simulink model "PIControlWithObserverR2_discrete_reorder_fixedpt"  (R2022b)
settings: Solver=VariableStepAuto  StartTime=0.0  StopTime=Tsim  FixedStep=dTMax  MaxStep=dTMax  RelTol=1e-3
values from neighbouring files (symbols this model uses):
  A = [A11 A12;A21 A22]    [VmPIWithObserverDriver_02Dec2022.m]    (also in observer_coeff.m)
  a1 = -1    [VmPIWithObserverDriver_02Dec2022.m]    (also in pi_controller_coeff.m = 0)
  a2 = 0    [VmPIWithObserverDriver_02Dec2022.m]
  Adp = LdC_inv*Ad    [VmPIWithObserverDriver_02Dec2022.m]    (also in observer_coeff.m = Adp)
  B = [B11;B21]    [VmPIWithObserverDriver_02Dec2022.m]    (also in observer_coeff.m)
  b0 = Gcd.num{1}(1)    [VmPIWithObserverDriver_02Dec2022.m]    (also in pi_controller_coeff.m = 1)
  b1 = Gcd.num{1}(2)    [VmPIWithObserverDriver_02Dec2022.m]    (also in pi_controller_coeff.m = 0)
  b2 = 0    [VmPIWithObserverDriver_02Dec2022.m]
  Bdp = Bdp/dac_scale    [VmPIWithObserverDriver_02Dec2022.m]    (also in observer_coeff.m = Bdp/dac_scale*total_scale)
  C = [C11 C12;C21 C22;C31 C32]    [VmPIWithObserverDriver_02Dec2022.m]    (also in observer_coeff.m)
  D = zeros(3,1)    [VmPIWithObserverDriver_02Dec2022.m]    (also in observer_coeff.m)
  dac_scale = 2^15    (= 32768)    [VmPIWithObserverDriver_02Dec2022.m]
  Im_scale = dn_per_amp    (= 246419753.086)    [VmPIWithObserverDriver_02Dec2022.m]
  Ldp = Ldp*[1/Im_scale, 0; 0, 1/VP1_scale]    [VmPIWithObserverDriver_02Dec2022.m]    (also in observer_coeff.m = Ldp*[1/Im_scale, 0; 0, 1/VP1_scale]*total_scale)
  N = 3    [VmPIWithObserverDriver_02Dec2022.m]
  Ts = 1/(MSPS*1e6)    (= 4e-07)    [VmPIWithObserverDriver_02Dec2022.m]
  VmDes = 0.025    [VmPIWithObserverDriver_02Dec2022.m]
  VP1_scale = dn_per_volt*10*1.7    (= 222822.4)    [VmPIWithObserverDriver_02Dec2022.m]
  x0 = [0.1*VmDes 0]'    [VmPIWithObserverDriver_02Dec2022.m]
settings Model: Creator=seco6437  LastModifiedBy=delg
settings DebuggingCC: UnconnectedInputMsg=warning  UnconnectedOutputMsg=warning  UnconnectedLineMsg=warning
settings ModelReferenceCC: EnableRefExpFcnMdlSchedulingChecks=on
settings RTWCC: DLArmComputeVersion=19.05

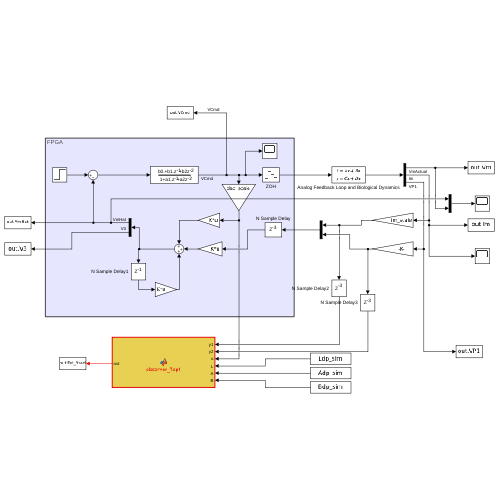
[thumbnail: Simulink's stored preview of the top-level diagram]
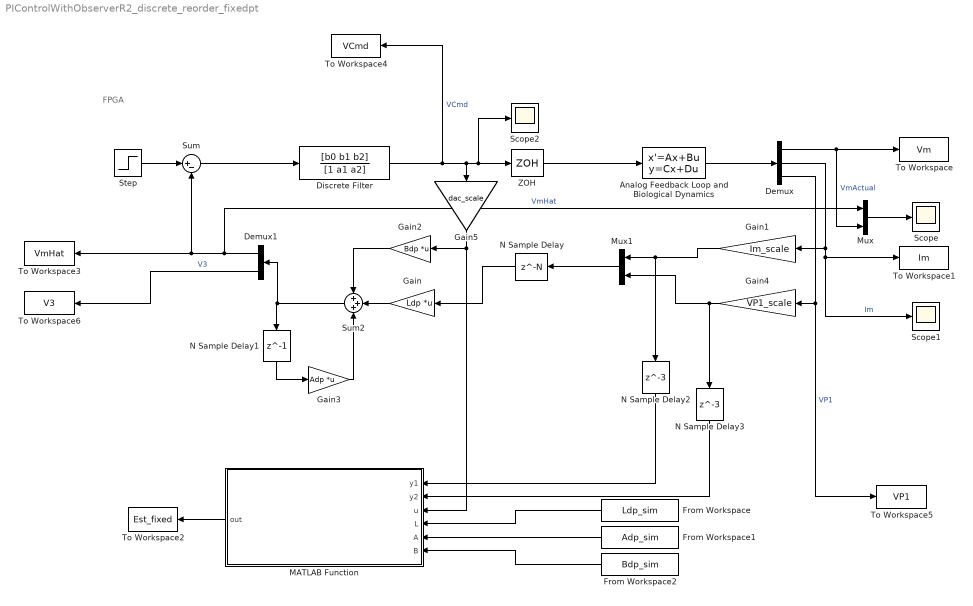
== system PIControlWithObserverR2_discrete_reorder_fixedpt ==
  note: FPGA
  Analog Feedback Loop and Biological Dynamics : StateSpace  A=A  B=B  C=C  D=D  InitialCondition=x0
  Demux : Demux  Outputs=3
  Demux1 : Demux  Outputs=2
  Discrete Filter : DiscreteFilter  Numerator=[b0 b1 b2]  Denominator=[1 a1 a2]  SampleTime=Ts
  From Workspace : FromWorkspace  VariableName=Ldp_sim  SampleTime=Ts  Interpolate=off  ZeroCross=off  OutputAfterFinalValue=Holding final value
  From Workspace1 : FromWorkspace  VariableName=Adp_sim  SampleTime=Ts  Interpolate=off  ZeroCross=off  OutputAfterFinalValue=Holding final value
  From Workspace2 : FromWorkspace  VariableName=Bdp_sim  SampleTime=Ts  Interpolate=off  ZeroCross=off  OutputAfterFinalValue=Setting to zero
  Gain : Gain  Gain=Ldp  Multiplication=Matrix(K*u)
  Gain1 : Gain  Gain=Im_scale
  Gain2 : Gain  Gain=Bdp  Multiplication=Matrix(K*u)
  Gain3 : Gain  Gain=Adp  Multiplication=Matrix(K*u)
  Gain4 : Gain  Gain=VP1_scale
  Gain5 : Gain  Gain=dac_scale
  MATLAB Function : MATLAB Function  TreatAsAtomicUnit=on
  Mux : Mux  Inputs=2
  Mux1 : Mux  Inputs=2
  N Sample Delay : Delay  DelayLength=N  SampleTime=Ts
  N Sample Delay1 : Delay  DelayLength=1  SampleTime=Ts
  N Sample Delay2 : Delay  DelayLength=3  SampleTime=Ts
  N Sample Delay3 : Delay  DelayLength=3  SampleTime=Ts
  Scope : Scope
  Scope1 : Scope
  Scope2 : Scope
  Step : Step  Time=0  After=VmDes  SampleTime=0
  Sum : Sum  Inputs=|+-
  Sum2 : Sum  Inputs=+++
  To Workspace : ToWorkspace  VariableName=Vm  SaveFormat=Timeseries  SampleTime=-1
  To Workspace1 : ToWorkspace  VariableName=Im  SaveFormat=Timeseries  SampleTime=-1
  To Workspace2 : ToWorkspace  VariableName=Est_fixed  SaveFormat=Timeseries  SampleTime=-1
  To Workspace3 : ToWorkspace  VariableName=VmHat  SaveFormat=Timeseries  SampleTime=-1
  To Workspace4 : ToWorkspace  VariableName=VCmd  SaveFormat=Timeseries  SampleTime=-1
  To Workspace5 : ToWorkspace  VariableName=VP1  SaveFormat=Timeseries  SampleTime=-1
  To Workspace6 : ToWorkspace  VariableName=V3  SaveFormat=Timeseries  SampleTime=-1
  ZOH : ZeroOrderHold  SampleTime=Ts
  wires:
  Analog Feedback Loop and Biological Dynamics/1 -> Demux/1
  Step/1 -> Sum/1
  N Sample Delay/1 -> Gain/1
  Sum2/1 -> N Sample Delay1/1, Demux1/1
  Gain2/1 -> Sum2/1
  Gain3/1 -> Sum2/3
  Gain/1 -> Sum2/2
  Sum/1 -> Discrete Filter/1
  ZOH/1 -> Analog Feedback Loop and Biological Dynamics/1
  Mux/1 -> Scope/1
  Demux1/1 -> Mux/1, To Workspace3/1, Sum/2  "VmHat"
  Demux1/2 -> To Workspace6/1  "V3"
  Demux/1 -> Mux/2, To Workspace/1  "VmActual"
  Demux/2 -> Scope1/1, To Workspace1/1, Gain1/1  "Im"
  Mux1/1 -> N Sample Delay/1
  Demux/3 -> To Workspace5/1, Gain4/1  "VP1"
  N Sample Delay1/1 -> Gain3/1
  MATLAB Function/1(out) -> To Workspace2/1
  From Workspace/1 -> MATLAB Function/4(L)
  From Workspace1/1 -> MATLAB Function/5(A)
  From Workspace2/1 -> MATLAB Function/6(B)
  Discrete Filter/1 -> To Workspace4/1, ZOH/1, Scope2/1, Gain5/1  "VCmd"
  Gain1/1 -> Mux1/1, N Sample Delay2/1
  Gain4/1 -> Mux1/2, N Sample Delay3/1
  Gain5/1 -> Gain2/1, MATLAB Function/3(u)
  N Sample Delay2/1 -> MATLAB Function/1(y1)
  N Sample Delay3/1 -> MATLAB Function/2(y2)

== matlab function PIControlWithObserverR2_discrete_reorder_fixedpt/MATLAB Function ==
  settings: updateMethod=DISCRETE  sampleTime=Ts
  data: y1 input; y2 input; u input; out output; L input; A input; B input
function out   = observer_fixpt(y1, y2, u, L, A, B)
    % inputs 
    % y1, y2, y3, L, A, B
    fm = get_fimath();

    y1 = fi(y1, 1, 16,0, fm);
    y2 = fi(y2, 1, 16,0, fm);
    u = fi(u, 1, 16,0, fm);

    persistent yest;
    if isempty(yest)
        yest = fi([0 0]', 1, 33, 32, fm);
%         yest = fi([0 0]', 1, 16, 17, fm);
    end

    Lm = fi(reshape(L,2,2), 1, 32, 50, fm);
    Am = fi(reshape(A,2,2), 1, 32, 24, fm);
    Bm = fi(reshape(B,2,1), 0, 32, 50, fm); % this is a Nx1 vector so reshape is uncessary 

    yest(:) = Am*yest + Bm*u + Lm*[fi(y1,1,16,0,fm) y2]'; 
    out = fi(yest, 1, 16, 15, fm);
end


function fm = get_fimath()
	fm = fimath('RoundingMethod', 'Floor',...
	     'OverflowAction', 'Wrap',...
	     'ProductMode','FullPrecision',...
	     'SumMode','FullPrecision');
end
